simulink model "harness"  (R2021b)
settings: Solver=VariableStepAuto  StartTime=0.0  StopTime=inf  FixedStep=1/10  RelTol=1e-3
libraries: simulink x1
settings Model: PacingRate=3  Creator=DAUIN-Win10  LastModifiedBy=gianlucalm

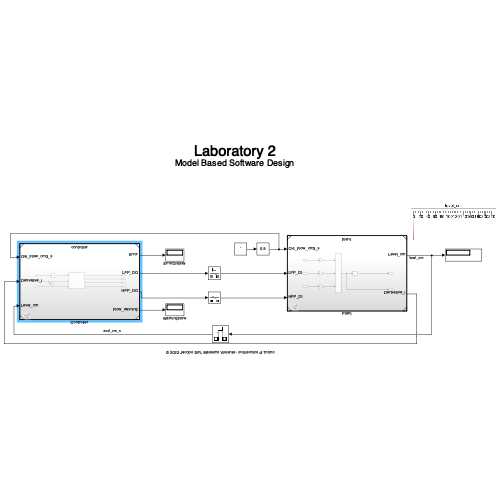
[thumbnail: Simulink's stored preview of the top-level diagram]
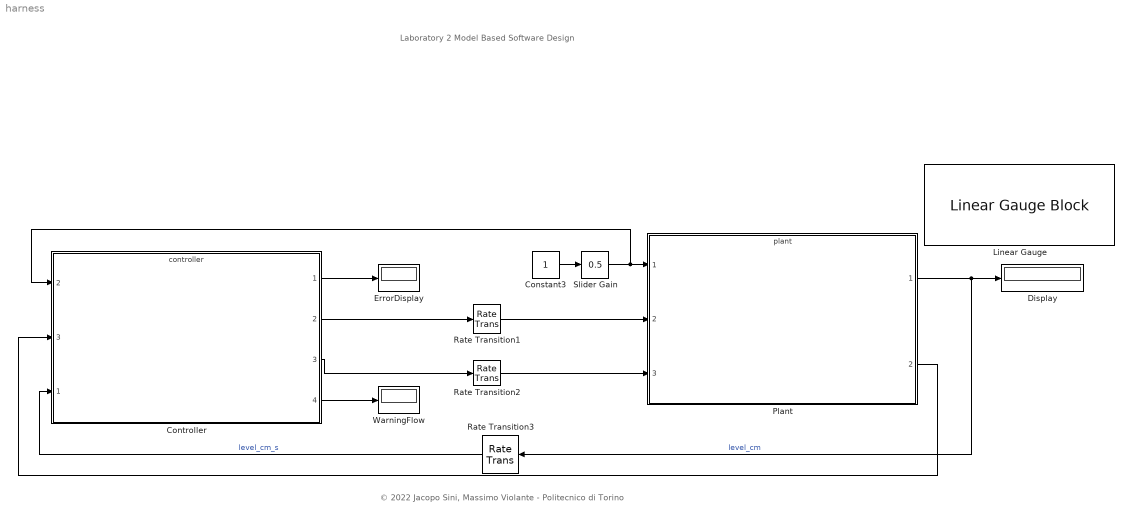
== system harness ==
  note: © 2022 Jacopo Sini, Massimo Violante - Politecnico di Torino
  note: Laboratory 2
      | Model Based Software Design
  Constant3 : Constant
  Controller : ModelReference  ModelNameDialog=controller  SimulationMode=Normal  ModelReferenceVersion=1.45
      settings: PortSchema="{\"entries\":[{\"content\":{\"sides\":[{\"content\":{\"connectorIds\":[\"In2\",\"In3\",\"In1\"]},\"type\":\"ConnectorPlacement.EquallySpacedRectSide\",\"uuid\":\"5e260b81-e1ce-497c-8572-ac5c2182ee27\"},{\"content\":{\"connectorIds\":[\"Out1\",\"Out2\",\"Out3\",\"Out4\"],\"side\":\"RIGHT\"},\"type\":\"ConnectorPlacement.EquallySpacedRectSide\",\"uuid\":\"4325f63c-e453-4c79-ab01-1476da99aa25\"},{\"content\":{\"connectorIds\":[],\"side\":\"TOP\"},\"type\":\"ConnectorPlacement.EquallySpacedRectSide\",\"uuid\":\"dba88bac-0f95-4a98-ba3b-c40df5616f56\"}]},\"type\":\"ConnectorPlacement.EquallySpacedConnector\",\"uuid\":\"6943e10d-f3b0-4fd8-a142-b6b49e651f90\"}],\"packageUris\":[\"http://schema.mathworks.com/mf0/Connector/R2020b\"],\"version\":\"1.0\"}"
  Display : Display
  ErrorDisplay : Display
  Linear Gauge : LinearGaugeBlock  ScaleMax=220
  Plant : ModelReference  ModelNameDialog=plant  SimulationMode=Normal  ModelReferenceVersion=1.10
  Rate Transition1 : RateTransition
  Rate Transition2 : RateTransition
  Rate Transition3 : RateTransition
  Slider Gain : simulink/Math Operations/Slider Gain  gain=0.5  low=0  high=1
  WarningFlow : Display
  wires:
  Controller/2 -> Rate Transition1/1
  Controller/3 -> Rate Transition2/1
  Plant/1 -> Rate Transition3/1, Display/1  "level_cm"
  Slider Gain/1 -> Controller/2, Plant/1
  Constant3/1 -> Slider Gain/1
  Controller/1 -> ErrorDisplay/1
  Rate Transition1/1 -> Plant/2
  Rate Transition2/1 -> Plant/3
  Rate Transition3/1 -> Controller/1  "level_cm_s"
  Plant/2 -> Controller/3
  Controller/4 -> WarningFlow/1
